simulink subsystem "Tether_dynamics_R2019B"  (R2022a)
settings: Solver=VariableStepAuto  StartTime=0.0  StopTime=10.0  RelTol=1e-3
undefined symbols (not defined in the file): ENVMT, T
settings Model: Creator=dylaneijkelhof  LastModifiedBy=kebl6571
settings SolverCC: AlgebraicLoopSolver=TrustRegion
settings DebuggingCC: UnconnectedInputMsg=warning  UnconnectedOutputMsg=warning  UnconnectedLineMsg=warning  SFMachineParentedDataDiag=warning

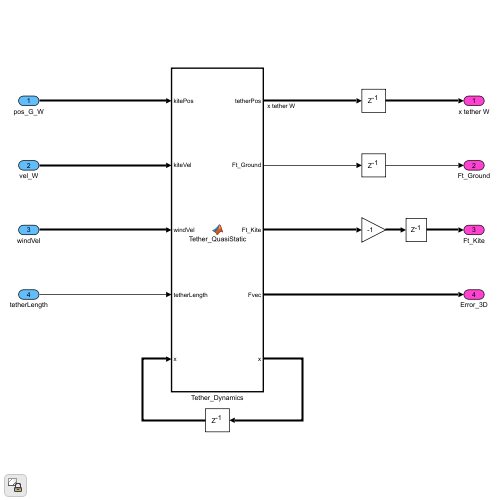
[thumbnail: Simulink's stored preview of the top-level diagram]
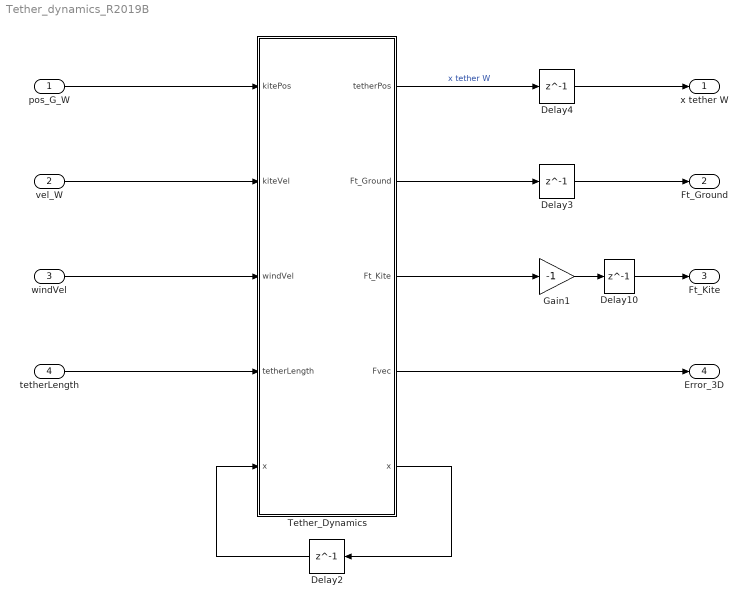
== system Tether_dynamics_R2019B ==
  pos_G_W : Inport
  vel_W : Inport  Port=2
  windVel : Inport  Port=3
  tetherLength : Inport  Port=4
  Delay10 : Delay  DelayLength=1  InitialCondition=zeros(3,1)
  Delay2 : Delay  DelayLength=1  InitialCondition=T.Tn_vect
  Delay3 : Delay  DelayLength=1
  Delay4 : Delay  DelayLength=1  InitialCondition=T.pos_p_init
  Gain1 : Gain  Gain=-1
  Tether_Dynamics : MATLAB Function  TreatAsAtomicUnit=on
  x tether W : Outport
  Ft_Ground : Outport  Port=2
  Ft_Kite : Outport  Port=3
  Error_3D : Outport  Port=4
  wires:
  Tether_Dynamics/4(Fvec) -> Error_3D/1
  vel_W/1 -> Tether_Dynamics/2(kiteVel)
  Tether_Dynamics/2(Ft_Ground) -> Delay3/1
  Tether_Dynamics/3(Ft_Kite) -> Gain1/1
  Tether_Dynamics/1(tetherPos) -> Delay4/1  "x tether W"
  pos_G_W/1 -> Tether_Dynamics/1(kitePos)
  windVel/1 -> Tether_Dynamics/3(windVel)
  Tether_Dynamics/5(x) -> Delay2/1
  Delay2/1 -> Tether_Dynamics/5("x ")
  Delay4/1 -> x tether W/1
  Delay3/1 -> Ft_Ground/1
  Gain1/1 -> Delay10/1
  Delay10/1 -> Ft_Kite/1
  tetherLength/1 -> Tether_Dynamics/4(tetherLength)

== matlab function Tether_dynamics_R2019B/Tether_Dynamics ==
  data: kitePos input; tetherPos output size=[3,T.np]; kiteVel input; windVel input; tetherLength input; x input; Ft_Ground output; Ft_Kite output; Fvec output; x output; ENVMT parameter; T parameter
% Copyright 2021 Delft University of Technology
%
% Licensed under the Apache License, Version 2.0 (the "License");
% you may not use this file except in compliance with the License.
% You may obtain a copy of the License at
%
%      http://www.apache.org/licenses/LICENSE-2.0
%
% Unless required by applicable law or agreed to in writing, software
% distributed under the License is distributed on an "AS IS" BASIS,
% WITHOUT WARRANTIES OR CONDITIONS OF ANY KIND, either express or implied.
% See the License for the specific language governing permissions and
% limitations under the License.

function [tetherPos, Ft_Ground, Ft_Kite, Fvec, x]= ...
    Tether_QuasiStatic(kitePos, kiteVel, windVel, tetherLength, x, ENVMT, T)
%#codegen

%Tether_QuasiStatic Trust-region dogleg nonlinear systems of equation
%   solver to determine the tether shape and forces.
%
%   Tether_QuasiStatic is based on the matlab implementation that 
%   solves a system of nonlinear equations using a dogleg
%   trust region approach.  The algorithm implemented is similar in nature
%   to the FORTRAN program HYBRD1 of J.J. More', B.S. Garbow and K.E. 
%   Hillstrom, User Guide for MINPACK 1, Argonne National Laboratory, 
%   Rept. ANL-80-74, 1980, which itself was based on the program CALFUN 
%   of M.J.D. Powell, A Fortran subroutine for solving systems of
%   nonlinear algebraic equations, Chap. 7 in P. Rabinowitz, ed.,
%   Numerical Methods for Nonlinear Algebraic Equations, Gordon and
%   Breach, New York, 1970.
%
%   Addapted by Ir. D. Eijkelhof (TU Delft) from 1990-2019 Matlab version 
%   The MathWorks, Inc.
% NOTE: From Matlab 2020b Matlab's Levenberg–Marquardt algorithm in the
% command "solve" can be directly used in codegen and might be
% faster. Due to availability of only matlab R2019B and lower, an own
% implementation had to be used in order the execute codegen.
%
% Syntax:  [tetherPos, Ft_Ground, Ft_Kite, Fvec, x]= ...
%     Tether_QuasiStatic(kitePos, kiteVel, windVel, tetherLength, x, ENVMT, T)
%
% NOTE: 'x' passed in and returned in column vector form.
%
% Throughout this routine 'x', 'F', 'xvec', 'xTrial', 'Fvec' and 'FTrial' are vectors.
%
% Inputs:
%    tetherPos  - Position vectors of tether particles
%    Ft_Ground  - Tether force magnitude at the ground station
%    Ft_Kite    - Tether force vector at the kite
%    Fvec       - Error between tether end and kite position (3D)
%    x          - Tether ground segment orientation and magnitude
%
% Outputs:
%    kitePos        - Kite position vector in wind reference frame
%    kiteVel        - Kite velocity vector in wind reference frame
%    windVel        - Wind velocity vector in wind reference frame
%    ENVMT          - Environmental parameters
%    tetherLength   - Reeled-out tether length determined by the winch
%    x              - Initial tether ground segment orientation and magnitude
%    T              - Tether dimensions and material properties
%
% Other m-files required: none
%
% Subfunctions: Objfunc    : Calculate difference between tether end and
%                            kite given tether ground segment orientation
%                            and magnitude.
%               testStop   : Test convergence criteria's
%               dogleg_tem : approximately solves trust region subproblem
%                            via a dogleg approach. 
%               lm_FD_J    : Determines the jacobian matrix by forward
%                            differencing
%
% MAT-files required: none
%
% Author: Dylan Eijkelhof, M.Sc.
% Delft University of Technology
% email address: d.eijkelhof@tudelft.nl  
% December 2019; Last revision: 16-March-2021

%------------- BEGIN CODE --------------
    
    [Fvec,T0,pj,~] = Objfunc(x,kitePos,kiteVel,windVel,tetherLength,ENVMT,T);
    
    xvec = x(:);         % vector representation of x
    % Convert values to full to avoid unnecessary sparse operation overhead
    % Initial x
    Fvec = full(Fvec); 
    
    % Set tolerances
    maxfunc     = 100*5;
    maxit       = 1000;
    tolf        = 1e-9;
    tolfunvalue = 1e-6;
    tolx        = 1e-6;
    tolobj      = 1e-6;
    
    nVar        = 3; % for codegen it worked better than numel(x)

    % Initialize local arrays.
    d           = zeros(nVar,1);

    % Initialize other trust region parameters.
    Delta       = 1e0;
    DeltaMax    = 1e10;
    eta1        = T.eta1;
    eta2        = T.eta2;
    alpha1      = T.alpha1;
    alpha2      = T.alpha2;

    % Extra initializations.
    iter        = 0;
    numFevals   = 1;

    stepAccept  = true;
    normd       = 0.0e0;
    objold      = 1.0e0;
    obj         = 0.5*(Fvec'*Fvec);  % Initial Fvec computed above

    numFDfevals = 0; %#ok<NASGU>
    JAC         = zeros(3,3); %#ok<PREALL> % pre-allocate derivative array

    %%%%%%%%%%%%%%%%%%%%%%% Calculate Jacobian at x0 %%%%%%%%%%%%%%%%%%
    [JAC,numFDfevals] = lm_FD_J(x, 0.1*ones(3,1),kitePos, kiteVel, ...
        windVel, tetherLength, ENVMT, T);

    % Increment the number of function evaluations with those used in the
    % finite difference calls.
    numFevals = numFevals + numFDfevals;

    grad = JAC'*Fvec;
    normgradinf = norm(grad,inf);

    % Test convergence at initial point.
    [done,~] = testStop(normgradinf,tolf,tolfunvalue,tolx,...
         stepAccept,iter,maxit,numFevals,maxfunc,Delta,normd,...
         obj,objold,d,xvec,tolobj,Fvec);

    % Beginning of main iteration loop.
    while ~done
    	iter = iter + 1;

    	% Compute step, d, using dogleg approach.
    	[d,quadObj,normd,normdscal] = ...
           dogleg(nVar,Fvec,JAC,grad,Delta);

        % Compute the model reduction given by d (pred).
        pred = -quadObj;

        % Compute the trial point, xTrial. Limit to positive value
        xTrial = xvec + d;
        if xTrial(3) < 0
            xTrial(3) = 1e-3;
        end

        % Evaluate nonlinear equations and objective at trial point.
        [F,T0,pj,~] = Objfunc(xTrial,kitePos,kiteVel,windVel,tetherLength,...
            ENVMT,T);
      
      
        numFevals = numFevals + 1;
        FTrial    = full(F(:)); % make FTrial a vector, convert to full
        objTrial  = 0.5*(FTrial'*FTrial); 

        % Compute the actual reduction given by xTrial (ared).
        ared      = obj - objTrial;

        % Compute ratio = ared/pred.
        if pred <= 0 % reject step
            ratio = 0;
        else
            ratio = ared/pred;
        end

        currTrialWellDefined = isfinite(objTrial);

        if ratio > eta1 && currTrialWellDefined % accept step.

            xvec    = xTrial; 
            objold  = obj; 
            obj     = objTrial;
            x(:)    = xvec; % update matrix representation
        
            %%%%%%%%%%%%%%%%%%%%%% Calculate New Jacobian %%%%%%%%%%%%%%%%%
            if iter == 1 || mod(iter,2*size(x,1))==0
                [JAC,numFDfevals] = lm_FD_J(x, 0.01*ones(3,1),kitePos, kiteVel, windVel, tetherLength, ENVMT, T);

                numFevals = numFevals + numFDfevals;
            else
                JAC = JAC + ((FTrial-Fvec-JAC*d)*d')/(d'*d);
            end
        
            Fvec        = FTrial; 
            grad        = JAC'*Fvec;
            normgradinf = norm(grad,inf);

            stepAccept  = true;
        else % reject step.
            stepAccept  = false;
        end 


        % Update trust region radius.
        if ~currTrialWellDefined
            % Shrink the trust region if any element of the function vector
            % at the new step is not defined (i.e. it's inf/NaN/complex). The
            % update for Delta in this case follows that in snls.
            Delta = min(normdscal/20,Delta/20);
        elseif ratio < eta1
            Delta = alpha2*normdscal;
        elseif ratio >= eta2
            Delta = max(Delta,alpha1*normdscal);
        end
        Delta = min(Delta,DeltaMax);

        % Check for termination.
        [done,~] = testStop(normgradinf,tolf,tolfunvalue,tolx,...
            stepAccept,iter,maxit,numFevals,maxfunc,Delta,normd,...
            obj,objold,d,xvec,tolobj,Fvec);
    end

    % Optimization is finished.  
    Ft_Ground   = x(3);
    Ft_Kite     = T0;
    tetherPos   = pj;
end

%%%%%%%%%%%%%%%%%%%%%%%%%%%%%%%%%%%%%%%%%%%%%%%%%%%%%%%%%%%%%%%
function [Fobj,T0,pj,p0] = Objfunc(stateVec,kitePos, kiteVel, windVel,...
                              tetherLength, ENVMT, T)
    Ns = size(windVel,2);       % number of masses
    Ls = tetherLength/(Ns+1);   % segment length
    mj = T.rho_t * Ls;          % segment mass

    p = kitePos;                % input aircraft position
    v = kiteVel;                % input aircraft velocity

    theta = stateVec(1);
    phi = stateVec(2);
    Tn = stateVec(3);

    omega_t = cross(p./(norm(p)^2),v);

    E = T.E;
    A = T.A;

    FT = zeros(3,Ns); % Tension forces
    Fd = zeros(3,Ns); % Drag forces
    pj = zeros(3,Ns); % Mass positions
    vj = zeros(3,Ns); % Mass velocities
    aj = zeros(3,Ns); % Mass accellerations

    % First element from ground station (Ns)
    FT(:,Ns) = Tn.*[sin(theta)* cos(phi); sin(phi); cos(theta)*cos(phi)];
    pj(:,Ns) = Ls.*[sin(theta)* cos(phi); sin(phi); cos(theta)*cos(phi)];
    vj(:,Ns) = dot(v,p./norm(p)) .* (p./norm(p)) + cross(omega_t,pj(:,Ns));
    aj(:,Ns) = cross(omega_t,cross(omega_t,pj(:,Ns)));
    
    % Drag calculation first element
    v_a_p = vj(:,Ns) - windVel(:,Ns);
    if all(abs(v_a_p)<1e-3)
        Fd(:,Ns) = [0;0;0];
    else
        v_a_p_t = dot((pj(:,Ns))/norm(pj(:,Ns)),v_a_p)*...
            ((pj(:,Ns))/norm(pj(:,Ns)));
        v_a_p_n = v_a_p - v_a_p_t;
        Fd(:,Ns) = -0.5 * ENVMT.rhos * Ls * T.d_tether * T.CD_tether * ...
            norm(v_a_p_n) * v_a_p_n; % particle drag
    end
    
    % All other segments and masses except for segment connected to the kite
    for i = Ns:-1:2
        if i == Ns
            FT(:,i-1) = (mj+0.5*mj).*aj(:,i) + FT(:,i) - Fd(:,i) + ...
                [0;0;(mj+0.5*mj)*ENVMT.g];
        else
            FT(:,i-1) = mj.*aj(:,i) + FT(:,i) - Fd(:,i) + [0;0;mj*ENVMT.g];
        end

        l_i_1 = (norm(FT(:,i-1))/(E*A) + 1)*Ls;
        
        pj(:,i-1) = pj(:,i) + l_i_1.*(FT(:,i-1)/norm(FT(:,i-1)));       
        vj(:,i-1) = dot(v,p./norm(p)) .* (p./norm(p)) + cross(omega_t,pj(:,i-1));
        aj(:,i-1) = cross(omega_t,cross(omega_t,pj(:,i-1)));
        
        % Drag calculation
        v_a_p = vj(:,i) - windVel(:,i);
        if all(abs(v_a_p)<1e-3)
            Fd(:,i-1) = [0;0;0];
        else
            v_a_p_t = dot((pj(:,i-1)-pj(:,i))/norm(pj(:,i-1)-pj(:,i)),v_a_p) * ...
                ((pj(:,i-1)-pj(:,i))/norm(pj(:,i-1)-pj(:,i)));
            v_a_p_n = v_a_p - v_a_p_t;
            Fd(:,i-1) = -0.5 * ENVMT.rhos * Ls * T.d_tether * T.CD_tether * ...
                norm(v_a_p_n) * v_a_p_n; % particle drag
        end
    end
    
    T0 = (mj+0.5*mj).*aj(:,1) + FT(:,1) - Fd(:,1) + [0;0;(mj+0.5*mj)*ENVMT.g];
    l_i_1 = (norm(T0)/(E*A) + 1)*Ls;
    p0 = pj(:,1) + l_i_1.*(T0/norm(T0));
    
    Fobj = p-p0;
end
%%%%%%%%%%%%%%%%%%%%%%%%%%%%%%%%%%%%%%%%%%%%%%%%%%%%%%%%%%%%%%%
function [done,EXITFLAG] = testStop(normgradinf,tolf,tolfunvalue,...
        tolx,stepAccept,iter,maxit,numFevals,maxfunc,Delta,normd,...
        obj,objold,d,xvec,tolobj,Fvec)
    %testStop checks the termination criteria for TRUSTNLEQN.

    done = false;
    EXITFLAG = 0;

    % Check termination criteria.

    if stepAccept && normgradinf < tolf
      EXITFLAG = 1;
      done = true;
      
    elseif iter > 1 && max(abs(d)./(abs(xvec)+1)) < max(tolx^2,eps)
       EXITFLAG = 2;
       done = true;
       
    elseif iter > 1 && stepAccept && normd < 0.9*Delta ...
                    && abs(objold-obj) < max(tolfunvalue^2,eps)*(1+abs(objold))
      EXITFLAG = 3;
      done = true;
      
    elseif iter > 1 && norm(Fvec) < tolobj
      EXITFLAG = 4;
      done = true;
      
    elseif Delta < 2*eps
      EXITFLAG = -3;
      done = true;
      
    elseif iter >= maxit
      EXITFLAG = 0;
      done = true;
      
    elseif numFevals >= maxfunc
      EXITFLAG = 0;
      done = true;
    end  
end
%%%%%%%%%%%%%%%%%%%%%%%%%%%%%%%%%%%%%%%%%%%%%%%%%%%%%%%%%%%%%%%
function [step,quadObj,normStep,normStepScal] = ...
    dogleg(nvar,F,JAC,grad,Delta)
%dogleg approximately solves trust region subproblem via a dogleg approach.
%
%   dogleg finds an approximate solution d to the problem:
%
%     min_d      f + g'd + 0.5*d'Bd
%
%     subject to ||Dd|| <= Delta
%
%   where g is the gradient of f, B is a Hessian approximation of f, D is a
%   diagonal scaling matrix and Delta is a given trust region radius.

%   Copyright 1990-2012 The MathWorks, Inc.
%   $Revision: 1.1.6.7 $  $Date: 2012/08/21 01:08:20 $

% NOTE: The scaling matrix D above is called scalMat in this routine.

% Compute scaled gradient and other scaled terms.
grad2 = grad;
normgradscal = norm(grad);

if normgradscal >= eps
    % First compute the Cauchy step (in scaled space).
    dCauchy = -(Delta/normgradscal)*grad;
    JACvec = JAC*grad2;
    denom = Delta*(JACvec'*JACvec);
    tauterm = normgradscal^3/denom;
    tauC = min(1,tauterm);
    dCauchy = tauC*dCauchy;
    
    % Compute quadratic objective at Cauchy point.
    JACvec = JAC*(dCauchy); 
    objCauchy = grad'*dCauchy + 0.5*(JACvec'*JACvec);   
    normdCauchy = min(norm(dCauchy),Delta);
else
    % Set Cauchy step to zero step and continue.
    objCauchy = 0;
    normdCauchy = 0;
    dCauchy = zeros(nvar,1);
end

if Delta - normdCauchy < eps
    % Take the Cauchy step if it is at the boundary of the trust region.
    step = dCauchy; quadObj = objCauchy;
else
    % Compute the Gauss-Newton step (in scaled space).
    
    dNewton = -JAC\F;
    
    if any(~isfinite(dNewton))
        % Take the Cauchy step if the Gauss-Newton step gives bad values.
        step = dCauchy; quadObj = objCauchy;
    else 
        normdNewt = norm(dNewton);
        if normdNewt <= Delta
            % Use the Newton direction as the trial step
            step = dNewton;
        else
            % Find the intersect point along dogleg path.
            Delta2 = Delta^2;
            normdCauchy2 = min(normdCauchy^2,Delta2);
            normdNewt2 = normdNewt^2;
            dCdN = dCauchy'*dNewton;
            dCdNdist2 = max((normdCauchy2+normdNewt2-2*dCdN),0);
            
            if dCdNdist2 == 0
                Lambda = 0;
            else
                % Stable method for solving 1-D quadratic
                a = 0.5*dCdNdist2;
                b = dCdN - normdCauchy2;
                c = 0.5*(normdCauchy2 - Delta2);
                q = -0.5*(b + sign(b)*sqrt(b^2 - 4*a*c));
                if b > 0
                    Lambda = c/q; 
                else
                    Lambda = q/a;
                end

                % Make sure we take a finite step,
                % (check for poorly scaled/infinite directions).
                if ~isfinite(Lambda)
                    Lambda = 0; % Take Cauchy step
                end
            end
            step = dCauchy + Lambda*(dNewton-dCauchy);
        end
        % Compute quadratic objective at trial point.
        JACvec = JAC*(step);
        quadObj = grad'*step + 0.5*(JACvec'*JACvec);
        
        % Compare Cauchy step and trial step (Newton or intersection)
        if objCauchy < quadObj
            step = dCauchy; quadObj = objCauchy;
        end
    end
end

% The step computed was the scaled step.  Unscale it.
normStepScal = norm(step);
normStep = norm(step);
end
 %%%%%%%%%%%%%%%%%%%%%%%%%%%%%%%%%%%%%%%%%%%%%%%%%%%%%%%%%%%%%%%
function [J,numFDfevals] = lm_FD_J(x, dp,kitePos, kiteVel, windVel, ...
                                tetherLength, ENVMT, T)

 m      = 3;                         % number of data points
 n      = 3;                         % number of parameters

 ps     = x; 
 J      = zeros(m,n); 
 del    = zeros(n,1);                % initialize Jacobian to Zero
 
 for j=1:n                           % START --- loop over all parameters

   del(j) = dp(j) * (1+abs(x(j)));   % parameter perturbation
   x(j)   = ps(j) + del(j);          % perturb parameter x(j)

   if del(j) ~= 0
     [y1,~,~,~] = Objfunc(x,kitePos, kiteVel, windVel, ...
         tetherLength, ENVMT, T);
     
     x(j) = ps(j) - del(j);
     [y,~,~,~] = Objfunc(x,kitePos, kiteVel, windVel, ...
         tetherLength, ENVMT, T);
     
     J(:,j) = (y1-y) ./ (2 .* del(j));
   end

   x(j) = ps(j);                     % restore x(j)

 end
 numFDfevals = 2;
                                     % END --- loop over all parameters
end
